simulink model "simulink_cosseno"  (R2023a)
settings: Solver=FixedStepAuto  StartTime=0.0  StopTime=10.0  FixedStep=1.0e-4  RelTol=1e-3
model workspace (MAT data in the model file):
  A = 10
  w = 5
settings Model: Creator=User  LastModifiedBy=Alexandre
settings SolverCC: AlgebraicLoopSolver=TrustRegion
settings DebuggingCC: UnconnectedInputMsg=warning  UnconnectedOutputMsg=warning  UnconnectedLineMsg=warning
settings ModelReferenceCC: EnableRefExpFcnMdlSchedulingChecks=on
settings RTWCC: DLArmComputeVersion=19.05

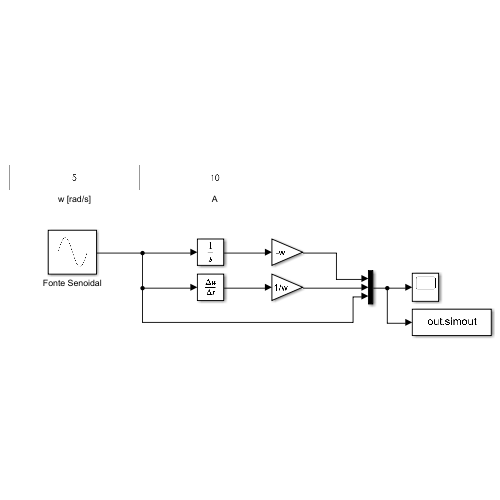
[thumbnail: Simulink's stored preview of the top-level diagram]
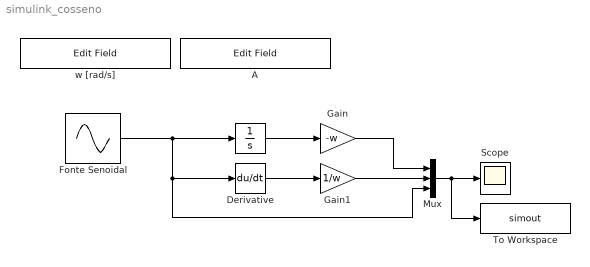
== system simulink_cosseno ==
  " " : Integrator  InitialCondition=-A/w
  A : EditField  LabelPosition=Hide  ShowInitialText=on  Alignment=Center
  Derivative : Derivative
  Fonte Senoidal : Sin  Amplitude=A  Frequency=w  SampleTime=0
  Gain : Gain  Gain=-w
  Gain1 : Gain  Gain=1/w
  Mux : Mux  Inputs=3
  Scope : Scope
  To Workspace : ToWorkspace  VariableName=simout  SampleTime=-1
  w [rad/s] : EditField  LabelPosition=Hide  ShowInitialText=on  Alignment=Center
  wires:
  Fonte Senoidal/1 -> Mux/3, Derivative/1, " "/1
  " "/1 -> Gain/1
  Derivative/1 -> Gain1/1
  Mux/1 -> To Workspace/1, Scope/1
  Gain1/1 -> Mux/2
  Gain/1 -> Mux/1
